simulink model "ADC_reader100sampling"  (R2025a)
settings: Solver=FixedStepAuto  StartTime=0.0  StopTime=inf  RelTol=1e-3  EnableMultiTasking=on
libraries: stm32f4xxblockslib x2, simulink x1
settings Model: STM32="{\"AnalogInput\":[{\"ID\":\"test_poten:20\"},{\"ID\":\"test_poten:28\"},{\"ID\":\"ADC_reader:28\"},{\"ID\":\"ADC_reader:20\"},{\"ID\":\"ADC_reader:14\"},{\"ID\":\"ADC_reader:11\"},{\"ID\":\"ADC_reader:8\"},{\"ID\":\"ADC_reader:5\"},{\"ID\":\"ADC_reader:1\"},{\"ID\":\"ADC_reader_simulink:28\"},{\"ID\":\"ADC_reader_simulink:38\"},{\"ID\":\"ADC_reader_simulink_PJ:28\"}],\"DigitalPortRead\":[{\"ID\":\"ADC_reader_simulink:42\"},{\"ID\":\"ADC_reader_simulink_PJ:42\"}]}"  Creator=ioonz  LastModifiedBy=tongl
settings OptimizationCC: DefaultParameterBehavior=Inlined  EnhancedBackFolding=on  PassReuseOutputArgsAs=Individual arguments  ZeroExternalMemoryAtStartup=off  ZeroInternalMemoryAtStartup=off  MaxStackSize=512  OptimizeBlockOrder=speed  DifferentSizesBufferReuse=on  OptimizationCustomize=off  EfficientTunableParamExpr=on
settings DebuggingCC: ParameterTunabilityLossMsg=error
settings HardwareCC: ProdBitPerPointer=32.0  ProdBitPerSizeT=32.0  ProdBitPerPtrDiffT=32.0  ProdLargestAtomicInteger=Long  ProdLargestAtomicFloat=Double  ProdWordSize=32.0  ProdLongLongMode=on  ProdHWDeviceType=ARM Compatible->ARM Cortex-M
settings SFSimCC: MATLABDynamicMemAlloc=off
settings RTWCC: SystemTargetFile=ert.tlc  HardwareBoard=STM32G4xx Based  TemplateMakefile=ert_default_tmf  Toolchain=GNU Tools for ARM Embedded Processors  Description=Embedded Coder
settings CodeAppCC: ForceParamTrailComments=on  IgnoreCustomStorageClasses=off  OperatorAnnotations=on  SimulinkDataObjDesc=on  SFDataObjDesc=on  InsertBlockDesc=on
settings ERTTargetCC: ExtModeTransport=3.0  ExtModeStaticAllocSize=2048.0  TargetLangStandard=C99 (ISO)  CodeReplacementLibrary=ARM Cortex-M

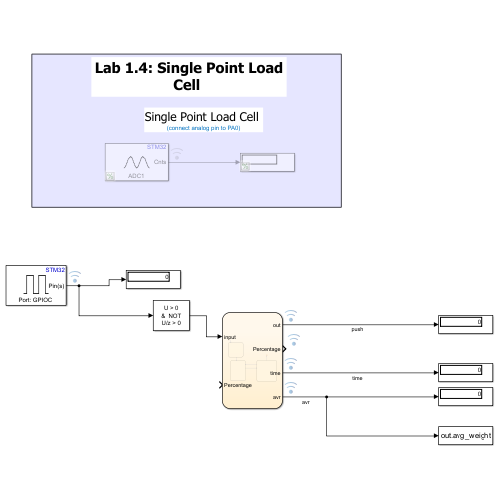
[thumbnail: Simulink's stored preview of the top-level diagram]
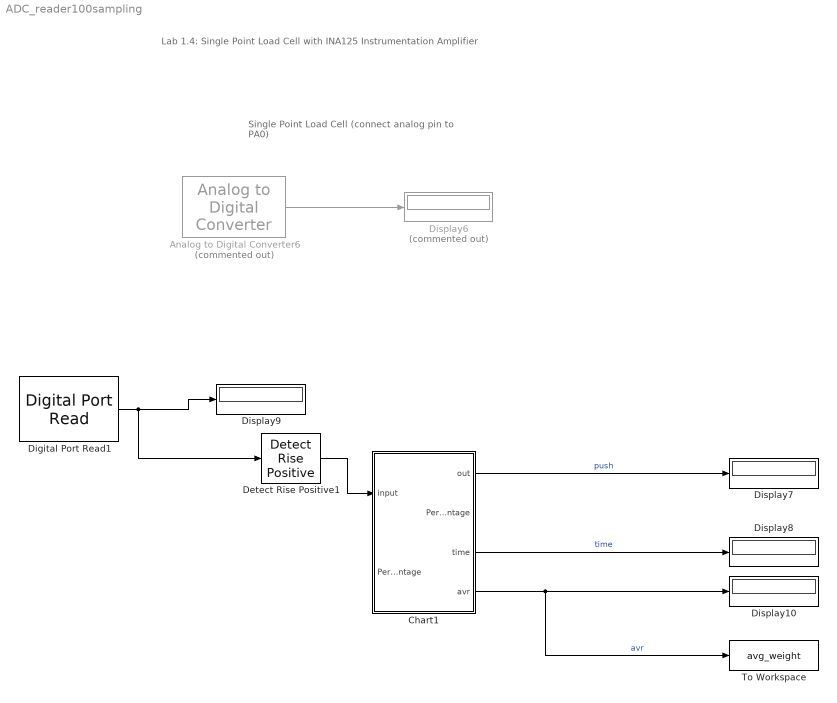
== system ADC_reader100sampling ==
  note: Single Point Load Cell
      | (connect analog pin to PA0)
  note: Lab 1.4: Single Point Load Cell
      | with INA125 Instrumentation Amplifier
  Analog to Digital Converter6 : stm32f4xxblockslib/Analog to Digital Converter  Commented=on  ADCModule=ADC1  ConversionGroup=Regular  TriggerMode=Trigger and read  NumberOfConversions=1  EnableBufferConv=off  BufferLength=1  OutputStatus=off  SampleTime=-1  EnableSimPort=off  hoistedMaskSrc=ECSoC/ECSimCodegen/Analog to Digital Converter
  Chart1 : Stateflow chart  TreatAsAtomicUnit=on
  Detect Rise Positive1 : simulink/Logic and Bit Operations/Detect Rise Positive  vinit=0  OutDataTypeStr=boolean
  Digital Port Read1 : stm32f4xxblockslib/Digital Port Read  PortName=GPIOC  PinNumber=[13]  ReadOperation=on  IOAsArray=on  SampleTime=-1  EnableSimPort=off  hoistedMaskSrc=ECSoC/ECSimCodegen/Digital Port Read
  Display{7..10} (4 alike) : Display
  Display6 : Display  Commented=on
  To Workspace : ToWorkspace  VariableName=avg_weight  SampleTime=-1
      settings: MaxDataPoints=2000  Save2DSignal=2-D array (concatenate along first dimension)
  wires:
  Analog to Digital Converter6/1 -> Display6/1
  Chart1/4(avr) -> To Workspace/1, Display10/1  "avr"
  Digital Port Read1/1 -> Detect Rise Positive1/1, Display9/1
  Chart1/1(out) -> Display7/1  "push"
  Chart1/3(time) -> Display8/1  "time"
  Detect Rise Positive1/1 -> Chart1/1(input)

== stateflow chart ADC_reader100sampling/Chart1 ==
  state Inital
    time = 0;
    out = 0;
    total = 0;
    avr = 0;
    round = 1;
  state HIGHT
    entry:
    out = 1;
    time = 0.01;
    avr = 0;
    during:
    time = time + 0.02
    Percentage = Percentage
    total = total + Percentage
    round = round + 1
  state Low
    entry:
    out = 0;
    avr = total/round
    total = 0;
    round = 0;
  (default) -> Inital
  HIGHT -> (junction 23) [order 2]
  Inital -> Low
  HIGHT -> Low [order 1] : [round >= 100]
  Low -> HIGHT : [input == 1]
  data: out output; Percentage output; input input; time output; Percentage input; avr output; total local; round local
